simulink model "control_rei_dh"  (R2021a)
settings: Solver=VariableStepAuto  StartTime=0.0  StopTime=20  RelTol=1e-3
values from neighbouring files (symbols this model uses):
  A_sys = [0 0     1  0 ... (first row only)    [control_dh.m]    (also in modelo_dh.m)
  B_sys = [0 ... (first row only)    [control_dh.m]    (also in modelo_dh.m)
  C_sys_cortada = [1 0 0 0]    [control_dh.m]
  K14 = Kss(1:4)    [control_dh.m]
  K5 = -Kss(5)    [control_dh.m]
libraries: simulink x1
settings Model: Creator=dherr  LastModifiedBy=dherr

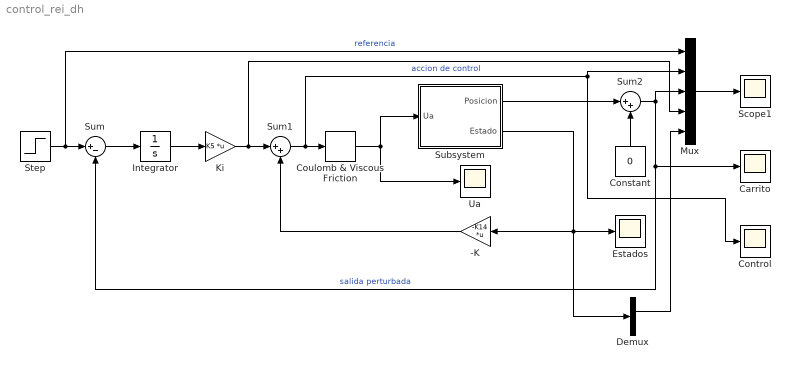
== system control_rei_dh ==
  -K : Gain  Gain=-K14  Multiplication=Matrix(K*u)
  Carrito : Scope
  Constant : Constant  Value=0
  Control : Scope
  Coulomb & Viscous Friction : simulink/Discontinuities/Coulomb & Viscous Friction  offset=[0.4]  gain=1
  Demux : Demux
  Estados : Scope
  Integrator : Integrator
  Ki : Gain  Gain=K5  Multiplication=Matrix(K*u)
  Mux : Mux  Inputs=5
  Scope1 : Scope
  Step : Step  Time=0  After=0.5  SampleTime=0
  Subsystem : Subsystem
  Sum : Sum  Inputs=|+-
  Sum1 : Sum  Inputs=|++
  Sum2 : Sum  Inputs=|++
  Ua : Scope
  wires:
  Coulomb & Viscous Friction/1 -> Ua/1, Subsystem/1(Ua)
  Subsystem/1(Posicion) -> Sum2/1
  Subsystem/2(Estado) -> Demux/1, -K/1, Estados/1
  Sum1/1 -> Control/1, Mux/2, Coulomb & Viscous Friction/1  "accion de control"
  -K/1 -> Sum1/2
  Ki/1 -> Mux/4, Sum1/1
  Integrator/1 -> Ki/1
  Sum/1 -> Integrator/1
  Step/1 -> Mux/1, Sum/1  "referencia"
  Sum2/1 -> Carrito/1, Sum/2, Mux/3  "salida perturbada"
  Mux/1 -> Scope1/1
  Constant/1 -> Sum2/2
  Demux/2 -> Mux/5

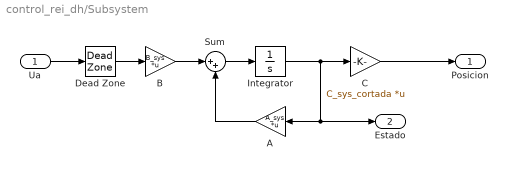
== system control_rei_dh/Subsystem ==
  Ua : Inport
  A : Gain  Gain=A_sys  Multiplication=Matrix(K*u)
  B : Gain  Gain=B_sys  Multiplication=Matrix(K*u)
  C : Gain  Gain=C_sys_cortada  Multiplication=Matrix(K*u)
  Dead Zone : DeadZone  UpperValue=0.6  SaturateOnIntegerOverflow=on
  Integrator : Integrator
  Sum : Sum  Inputs=|++
  Posicion : Outport
  Estado : Outport  Port=2
  wires:
  A/1 -> Sum/2
  Dead Zone/1 -> B/1
  Integrator/1 -> Estado/1, A/1, C/1
  Ua/1 -> Dead Zone/1
  B/1 -> Sum/1
  C/1 -> Posicion/1
  Sum/1 -> Integrator/1
